simulink model "general_charger_2_cc_cv_test"  (R2013a)
settings: Solver=ode23  StartTime=0  StopTime=1.5  RelTol=1e-3
PreLoadFcn:
  | Ts =5e-6;
values from neighbouring files (symbols this model uses):
  ac_volt = 169    [charger_init.m]    (also in charger_init_simpl.m)
  acdc_on_time = 0.2    [charger_init.m]    (also in charger_init_simpl.m = 0)
  Cdc = 2e-3    (= 0.002)    [charger_init.m]    (also in charger_init_simpl.m)
  dcAd = dcinvexp*(eye(dcnstates) + (Ts/2)*dcAc)    [charger_init.m]    (also in charger_init_simpl.m)
  dcBd = dcinvexp*dcBc    [charger_init.m]    (also in charger_init_simpl.m)
  dcCd = dcCc*dcinvexp*Ts    [charger_init.m]    (also in charger_init_simpl.m)
  dcDd = dcCc*dcinvexp*dcBc*(Ts/2) + dcDc    [charger_init.m]    (also in charger_init_simpl.m)
  ESLCd = 0.1e-9    (= 1e-10)    [charger_init.m]    (also in charger_init_simpl.m)
  ESRCd = 70e-3    (= 0.07)    [charger_init.m]    (also in charger_init_simpl.m)
  ESRLdcdc = 0.1    [charger_init.m]    (also in charger_init_simpl.m)
  ESRLin = 0.2    [charger_init.m]    (also in charger_init_simpl.m = 0.1)
  Ldcdc = 1.3e-3    (= 0.0013)    [charger_init.m]    (also in charger_init_simpl.m = 0.0014)
  Lin = 1.5e-3    (= 0.0015)    [charger_init.m]    (also in charger_init_simpl.m = 0.001)
  P = 1.92e3    (= 1920)    [charger_init.m]    (also in charger_init_simpl.m)
  Q = 0    [charger_init.m]    (also in charger_init_simpl.m)
  ramp = (dc_volt - Vdcmin)/(acdc_ramp_end_time)    (= 202)    [charger_init.m]    (also in charger_init_simpl.m = (dc_volt - Vdcmin)/(acdc_ramp_end_time))
  Rbatt = 0.20    (= 0.2)    [charger_init.m]    (also in charger_init_simpl.m = 0.1)
  switch_Ts = 5e-5    (= 5e-05)    [charger_init.m]    (also in charger_init_simpl.m)
  sys_Ts = 5e-6    (= 5e-06)    [charger_init.m]    (also in charger_init_simpl.m)
  Vdcmin = ac_volt + 10    (= 179)    [charger_init.m]    (also in charger_init_simpl.m)
  voc = 105    [charger_init.m]    (also in charger_init_simpl.m)
undefined symbols (not defined in the file or in its folder): CESR, cpi
undefined symbols (not defined in the file): active_power_on, Ad, Bd, Cd, dc_volt, dcdc_cc_ref, dcdc_cv_ref, dcdc_iki, dcdc_ikp, dcdc_on, dcdc_vki, dcdc_vkp, Dd, dq_id_ki, dq_id_kp, dq_iq_ki, dq_iq_kp, dq_vdc_ki, dq_vdc_kp, dqQ_ki, dqQ_kp, P_ki, P_kp, pi_iac_ki, pi_iac_kp, pi_vdc_ki, pi_vdc_kp, piQ_ki, piQ_kp, pr_iac_kp, pr_pr_ki, pr_pr_kp, pr_vdc_ki, pr_vdc_kp, reactive_power_on
libraries: simulink_extras x165, powerlib x61, simulink x35, powerlib_meascontrol x11
(part 3 of 7)

== system general_charger_2_cc_cv_test/control_stage/AC//DC Control/PR Controller ==
  inputs : Inport
  Add2 : Sum  Inputs=-+
  Add3 : Sum  Inputs=+-
  Constant2 : Constant  Value=vdc_ref
  Constant3 : Constant  Value=ac_peak
  Demux1 : Demux  Outputs=3
  Divide1 : Product  Inputs=/*
  PI Reactive Power Controller : Subsystem
  PI2 : Subsystem  mask{ki=vdc_ki, kp=vdc_kp, Ts_pi=Ts, int_sat_up=500, int_sat_low=-500, pi_sat_up=500, pi_sat_low=-500}
      mask prompts: ki "Integral Gain"; kp "Proportional Gain"; Ts_pi "Sample Time"; int_sat_up "Integral Saturation Upper"; int_sat_low "Integral Saturation Lower"; pi_sat_up "PI Controller Saturation Upper"; pi_sat_low "PI Controller Saturation Lower"
      mask Display: disp('PI')
  PR Controller : Subsystem
  Product2 : Product  RndMeth=Zero
  Scope : Scope  NumInputPorts=2
      settings: YMin=-1~-1  YMax=1~1  SaveName=ScopeData4
  Step1 : Step  Time=1/60  Before=1  After=0  SampleTime=0
  Switch3 : Switch  Threshold=0.5
  v_cont : Outport
  wires:
  Constant2/1 -> Add2/2
  Demux1/2 -> Add2/1  "vdc"
  Add2/1 -> PI2/1(in)
  PI2/1(out) -> Product2/2
  Demux1/1 -> Divide1/2  "vac"
  Constant3/1 -> Divide1/1
  Product2/1 -> Add3/1
  Demux1/3 -> Add3/2  "iac"
  Add3/1 -> PR Controller/2(iac error)
  PR Controller/1(output) -> v_cont/1
  Divide1/1 -> Switch3/1, PI Reactive Power Controller/1(vac in)
  PI Reactive Power Controller/1(vac shifted) -> Switch3/3
  Step1/1 -> Switch3/2
  inputs/1 -> Demux1/1
  Switch3/1 -> Product2/1, PR Controller/1(vac)

== system general_charger_2_cc_cv_test/control_stage/DC//DC Control/DC Pass Filter (1st Order)1 ==
  u[k] : Inport
  A : Gain  Gain=dcAd
  B : Gain  Gain=dcBd
  C : Gain  Gain=dcCd
  D : Gain  Gain=dcDd
  Delay : Delay  DelayLength=1  InitialCondition=0  SampleTime=5e-5
  Sum : Sum  Inputs=|++
  Sum1 : Sum  Inputs=|++
  y[k] : Outport
  wires:
  B/1 -> Sum/1
  u[k]/1 -> D/1, B/1
  Sum1/1 -> y[k]/1
  Delay/1 -> A/1, C/1
  Sum/1 -> Delay/1
  D/1 -> Sum1/1
  A/1 -> Sum/2
  C/1 -> Sum1/2

== system general_charger_2_cc_cv_test/control_stage/DC//DC Control/PI1 ==
  in : Inport
  Add1 : Sum
  Add2 : Sum
  Constant : Constant  Value=0
  Ki : Gain  Gain=ki
  Kp : Gain  Gain=kp
  Step : Step  Time=pi_on  SampleTime=0
  Switch : Switch  Threshold=0.5
  Tappe : simulink/Discrete/Tapped Delay  vinit=0.0  samptime=Ts_pi  NumDelays=1  DelayOrder=Oldest  includeCurrent=off
  Ts : Gain  Gain=Ts_pi
  integral saturation : Saturate  UpperLimit=int_sat_up  LowerLimit=int_sat_low  SampleTime=Ts_pi
  pi controller saturation : Saturate  UpperLimit=pi_sat_up  LowerLimit=pi_sat_low  SampleTime=Ts_pi
  out : Outport
  wires:
  Ts/1 -> Ki/1
  Add1/1 -> integral saturation/1  "vdc_int_pi"
  Kp/1 -> Add2/2  "vdc_kp_pi"
  pi controller saturation/1 -> out/1
  Tappe/1 -> Add1/1
  Ki/1 -> Add1/2
  integral saturation/1 -> Add2/1, Tappe/1
  Step/1 -> Switch/2
  Constant/1 -> Switch/3
  Add2/1 -> pi controller saturation/1  "vdc_pi"
  Switch/1 -> Kp/1, Ts/1
  in/1 -> Switch/1  "vdc_error"

== system general_charger_2_cc_cv_test/control_stage/DC//DC Control/PI2 ==
  in : Inport
  Add1 : Sum
  Add2 : Sum
  Constant : Constant  Value=0
  Constant1 : Constant  Value=0
  Ki : Gain  Gain=ki
  Kp : Gain  Gain=kp
  Logical Operator : Logic  Operator=XOR  IconShape=distinctive  AllPortsSameDT=off  OutDataTypeStr=boolean
  Scope : Scope
      settings: SaveName=ScopeData21
  Step : Step  Time=pi_on  SampleTime=0
  Step1 : Step  Time=pturn_on  SampleTime=switch_Ts
  Step2 : Step  Time=pturn_on + switch_Ts  SampleTime=switch_Ts
  Switch : Switch  Threshold=0.5
  Switch1 : Switch  Threshold=0.5
  Tappe : simulink/Discrete/Tapped Delay  vinit=0.0  samptime=Ts_pi  NumDelays=1  DelayOrder=Oldest  includeCurrent=off
  Ts : Gain  Gain=Ts_pi
  integral saturation : Saturate  UpperLimit=int_sat_up  LowerLimit=int_sat_low  SampleTime=Ts_pi
  pi controller saturation : Saturate  UpperLimit=pi_sat_up  LowerLimit=pi_sat_low  SampleTime=Ts_pi
  out : Outport
  wires:
  Ts/1 -> Ki/1
  Add1/1 -> integral saturation/1  "vdc_int_pi"
  Kp/1 -> Add2/2  "vdc_kp_pi"
  pi controller saturation/1 -> out/1
  Ki/1 -> Add1/2
  integral saturation/1 -> Add2/1, Tappe/1
  Step/1 -> Switch/2
  Constant/1 -> Switch/3
  Add2/1 -> pi controller saturation/1  "vdc_pi"
  Switch/1 -> Kp/1, Ts/1
  in/1 -> Switch/1  "vdc_error"
  Tappe/1 -> Switch1/3
  Switch1/1 -> Add1/1
  Logical Operator/1 -> Switch1/2, Scope/1
  Step2/1 -> Logical Operator/2
  Step1/1 -> Logical Operator/1
  Constant1/1 -> Switch1/1

== system general_charger_2_cc_cv_test/control_stage/DC//DC Control/PI3 ==
  in : Inport
  Add1 : Sum
  Add2 : Sum
  Constant : Constant  Value=0
  Ki : Gain  Gain=ki
  Kp : Gain  Gain=kp
  Step : Step  Time=pi_on  SampleTime=0
  Switch : Switch  Threshold=0.5
  Tappe : simulink/Discrete/Tapped Delay  vinit=0.0  samptime=Ts_pi  NumDelays=1  DelayOrder=Oldest  includeCurrent=off
  Ts : Gain  Gain=Ts_pi
  integral saturation : Saturate  UpperLimit=int_sat_up  LowerLimit=int_sat_low  SampleTime=Ts_pi
  pi controller saturation : Saturate  UpperLimit=pi_sat_up  LowerLimit=pi_sat_low  SampleTime=Ts_pi
  out : Outport
  wires:
  Ts/1 -> Ki/1
  Add1/1 -> integral saturation/1  "vdc_int_pi"
  Kp/1 -> Add2/2  "vdc_kp_pi"
  pi controller saturation/1 -> out/1
  Tappe/1 -> Add1/1
  Ki/1 -> Add1/2
  integral saturation/1 -> Add2/1, Tappe/1
  Step/1 -> Switch/2
  Constant/1 -> Switch/3
  Add2/1 -> pi controller saturation/1  "vdc_pi"
  Switch/1 -> Kp/1, Ts/1
  in/1 -> Switch/1  "vdc_error"

== system general_charger_2_cc_cv_test/control_stage/DC//DC Control/PI4 ==
  in : Inport
  Add1 : Sum
  Add2 : Sum
  Constant : Constant  Value=0
  Ki : Gain  Gain=ki
  Kp : Gain  Gain=kp
  Step : Step  Time=pi_on  SampleTime=0
  Switch : Switch  Threshold=0.5
  Tappe : simulink/Discrete/Tapped Delay  vinit=0.0  samptime=Ts_pi  NumDelays=1  DelayOrder=Oldest  includeCurrent=off
  Ts : Gain  Gain=Ts_pi
  integral saturation : Saturate  UpperLimit=int_sat_up  LowerLimit=int_sat_low  SampleTime=Ts_pi
  pi controller saturation : Saturate  UpperLimit=pi_sat_up  LowerLimit=pi_sat_low  SampleTime=Ts_pi
  out : Outport
  wires:
  Ts/1 -> Ki/1
  Add1/1 -> integral saturation/1  "vdc_int_pi"
  Kp/1 -> Add2/2  "vdc_kp_pi"
  pi controller saturation/1 -> out/1
  Tappe/1 -> Add1/1
  Ki/1 -> Add1/2
  integral saturation/1 -> Add2/1, Tappe/1
  Step/1 -> Switch/2
  Constant/1 -> Switch/3
  Add2/1 -> pi controller saturation/1  "vdc_pi"
  Switch/1 -> Kp/1, Ts/1
  in/1 -> Switch/1  "vdc_error"

== system general_charger_2_cc_cv_test/control_stage/DC//DC Control/half bridge control ==
  v_cont : Inport
  Add1 : Sum
  Constant : Constant
  Constant1 : Constant  Value=0
  Constant2 : Constant  Value=2500
  Constant3 : Constant  Value=0
  Logical Operator : Logic  Operator=NOT  IconShape=distinctive  AllPortsSameDT=off  OutDataTypeStr=boolean
  Product2 : Product  RndMeth=Zero
  Relational Operator1 : RelationalOperator  OutDataTypeStr=boolean
  Repeating Sequence2 : simulink/Sources/Repeating Sequence  rep_seq_t=[0 25e-6 50e-6]  rep_seq_y=[0 2500 0]
  Saturation1 : Saturate  UpperLimit=2500  LowerLimit=0
  Step : Step  Time=turn_on  SampleTime=0
  Step1 : Step  Time=turn_on  SampleTime=0
  Switch : Switch  Threshold=0.5
  Switch1 : Switch  Threshold=0.5
  tag scope: E=global, F=global
  wires:
  v_cont/1 -> Product2/2
  Repeating Sequence2/1 -> Relational Operator1/2
  Constant2/1 -> Product2/1
  Saturation1/1 -> Relational Operator1/1
  Product2/1 -> Add1/2
  Constant1/1 -> Add1/1
  Add1/1 -> Saturation1/1
  Logical Operator/1 -> [F]
  Step/1 -> Switch/2
  Constant/1 -> Switch/3
  Step1/1 -> Switch1/2
  Constant3/1 -> Switch1/3
  Relational Operator1/1 -> Switch/1, Switch1/1
  Switch/1 -> Logical Operator/1
  Switch1/1 -> [E]

== system general_charger_2_cc_cv_test/Measurements/Power and angle calculations/AB-DQ Transform/Iab_dq ==
  A : Inport
  wt : Inport  Port=2
  phi : Inport  Port=3
  Add1 : Sum  Inputs=-+
  Add2 : Sum
  Delay : Delay  DelayLength=RSpC  SampleTime=abdq_Ts
  Gain : Gain  Gain=-1
  Id Discretization Error Correction : Subsystem
  Iq Discretization Error Correction : Subsystem
  Product{1..4} (4 alike) : Product  RndMeth=Zero
  Scope : Scope  NumInputPorts=4
      settings: YMin=3.5~3.5~-17.5~-17.5  YMax=10~10~2.5~2.5  SaveName=ScopeData13
  Trigonometric Function : Trigonometry
  Trigonometric Function1 : Trigonometry  Operator=cos
  Unit Delay : UnitDelay  SampleTime=switch_Ts
  D : Outport
  Q : Outport  Port=2
  wires:
  Trigonometric Function/1 -> Product1/1, Product2/1
  Product1/1 -> Add2/2
  Product4/1 -> Add2/1
  Product2/1 -> Add1/1
  A/1 -> Delay/1, Product4/1, Product2/2
  Trigonometric Function1/1 -> Product4/2, Product3/1
  Product3/1 -> Add1/2
  Delay/1 -> Product1/2, Product3/2  "B"
  wt/1 -> [theta], Trigonometric Function1/1, Trigonometric Function/1
  Add2/1 -> Scope/2, Id Discretization Error Correction/3(D)  "Vd"
  Add1/1 -> Scope/3, Iq Discretization Error Correction/2(Q)
  [theta] -> Iq Discretization Error Correction/3(wt)
  [theta] -> Id Discretization Error Correction/2(wt)
  Id Discretization Error Correction/1(Id_corr) -> Scope/1, D/1
  Iq Discretization Error Correction/1(Iq_corr) -> Scope/4, Q/1
  phi/1 -> Gain/1
  Unit Delay/1 -> Iq Discretization Error Correction/1(phi), Id Discretization Error Correction/4(phi)
  Gain/1 -> Unit Delay/1
  [Ipeak] -> Iq Discretization Error Correction/4(A)
  [Ipeak] -> Id Discretization Error Correction/1(A)

== system general_charger_2_cc_cv_test/Measurements/Power and angle calculations/AB-DQ Transform/Vab_dq ==
  note: PLL based on dq frame control
      | input signal is assumed to be 60 Hz
      | and sample time is 50e-6
  signal_in : Inport
  AB->DQ : Subsystem  mask{abdq_f=pll_f, abdq_Ts=pll_Ts}
      mask prompts: abdq_f "frequency"; abdq_Ts "Sample Time"
      mask init:
      | SpC=1/abdq_f/4/abdq_Ts;
      | RSpC=ceil(SpC);
  Constant1 : Constant  Value=0
  Constant3 : Constant  Value=2*pi*pll_f
  PI1 : Subsystem  mask{ki=1, kp=0, Ts_pi=pll_Ts, int_sat_up=inf, int_sat_low=-inf, pi_sat_up=inf, pi_sat_low=-inf}
      mask prompts: ki "Integral Gain"; kp "Proportional Gain"; Ts_pi "Sample Time"; int_sat_up "Integral Saturation Upper"; int_sat_low "Integral Saturation Lower"; pi_sat_up "PI Controller Saturation Upper"; pi_sat_low "PI Controller Saturation Lower"
      mask Display: disp('PI')
  PI4 : Subsystem  mask{ki=pll_ki, kp=pll_kp, Ts_pi=pll_Ts, int_sat_up=inf, int_sat_low=-inf, pi_sat_up=inf, pi_sat_low=-inf}
      mask prompts: ki "Integral Gain"; kp "Proportional Gain"; Ts_pi "Sample Time"; int_sat_up "Integral Saturation Upper"; int_sat_low "Integral Saturation Lower"; pi_sat_up "PI Controller Saturation Upper"; pi_sat_low "PI Controller Saturation Lower"
      mask Display: disp('PI')
  Sum : Sum  Inputs=|-+
  Sum2 : Sum  Inputs=|-+
  angle_out : Outport
  D : Outport  Port=2
  Q : Outport  Port=3
  wires:
  Constant1/1 -> Sum/2
  Sum/1 -> PI4/1(in)
  PI1/1(out) -> angle_out/1, AB->DQ/2(wt)
  Constant3/1 -> Sum2/2
  PI4/1(out) -> Sum2/1
  AB->DQ/2(Q) -> Q/1, Sum/1
  signal_in/1 -> AB->DQ/1(A)
  AB->DQ/1(D) -> D/1
  Sum2/1 -> PI1/1(in)  "pll_int_error"

== system general_charger_2_cc_cv_test/Measurements/Power and angle calculations/RMS1/PI3 ==
  in : Inport
  Add1 : Sum
  Add2 : Sum
  Ki : Gain  Gain=ki
  Kp : Gain  Gain=kp
  Tappe : simulink/Discrete/Tapped Delay  vinit=0.0  samptime=Ts_pi  NumDelays=1  DelayOrder=Oldest  includeCurrent=off
  Ts : Gain  Gain=Ts_pi
  integral saturation : Saturate  UpperLimit=int_sat_up  LowerLimit=int_sat_low  SampleTime=Ts_pi
  pi controller saturation : Saturate  UpperLimit=pi_sat_up  LowerLimit=pi_sat_low  SampleTime=Ts_pi
  out : Outport
  wires:
  Ts/1 -> Ki/1
  in/1 -> Kp/1, Ts/1  "vdc_error"
  Add1/1 -> integral saturation/1  "vdc_int_pi"
  Kp/1 -> Add2/2  "vdc_kp_pi"
  pi controller saturation/1 -> out/1
  Tappe/1 -> Add1/1
  Add2/1 -> pi controller saturation/1  "vdc_pi"
  Ki/1 -> Add1/2
  integral saturation/1 -> Add2/1, Tappe/1

== system general_charger_2_cc_cv_test/Measurements/Power and angle calculations/RMS4/PI3 ==
  in : Inport
  Add1 : Sum
  Add2 : Sum
  Ki : Gain  Gain=ki
  Kp : Gain  Gain=kp
  Tappe : simulink/Discrete/Tapped Delay  vinit=0.0  samptime=Ts_pi  NumDelays=1  DelayOrder=Oldest  includeCurrent=off
  Ts : Gain  Gain=Ts_pi
  integral saturation : Saturate  UpperLimit=int_sat_up  LowerLimit=int_sat_low  SampleTime=Ts_pi
  pi controller saturation : Saturate  UpperLimit=pi_sat_up  LowerLimit=pi_sat_low  SampleTime=Ts_pi
  out : Outport
  wires:
  Ts/1 -> Ki/1
  in/1 -> Kp/1, Ts/1  "vdc_error"
  Add1/1 -> integral saturation/1  "vdc_int_pi"
  Kp/1 -> Add2/2  "vdc_kp_pi"
  pi controller saturation/1 -> out/1
  Tappe/1 -> Add1/1
  Add2/1 -> pi controller saturation/1  "vdc_pi"
  Ki/1 -> Add1/2
  integral saturation/1 -> Add2/1, Tappe/1

== system general_charger_2_cc_cv_test/Measurements/Power and angle calculations/discrete low pass filter1/Ad(1,1) ==
  in : Inport
  Constant1 : Constant  Value=variable
  Product1 : Product
  q rounder16 : Subsystem  mask{q=nQ, range=maxRange}
      mask prompts: q "q value"; range "q range"
  out : Outport
  wires:
  q rounder16/1(out) -> Product1/1
  Constant1/1 -> q rounder16/1(in)
  Product1/1 -> out/1
  in/1 -> Product1/2

== system general_charger_2_cc_cv_test/Measurements/Power and angle calculations/discrete low pass filter1/Ad(1,2) ==
  in : Inport
  Constant1 : Constant  Value=variable
  Product1 : Product
  q rounder16 : Subsystem  mask{q=nQ, range=maxRange}
      mask prompts: q "q value"; range "q range"
  out : Outport
  wires:
  q rounder16/1(out) -> Product1/1
  Constant1/1 -> q rounder16/1(in)
  Product1/1 -> out/1
  in/1 -> Product1/2

== system general_charger_2_cc_cv_test/Measurements/Power and angle calculations/discrete low pass filter1/Ad(1,3) ==
  in : Inport
  Constant1 : Constant  Value=variable
  Product1 : Product
  Scope1 : Scope  NumInputPorts=2
      settings: YMin=-5~-5  YMax=5~5
  q rounder16 : Subsystem  mask{q=nQ, range=maxRange}
      mask prompts: q "q value"; range "q range"
  out : Outport
  wires:
  q rounder16/1(out) -> Product1/1, Scope1/2
  Constant1/1 -> Scope1/1, q rounder16/1(in)
  Product1/1 -> out/1
  in/1 -> Product1/2

== system general_charger_2_cc_cv_test/Measurements/Power and angle calculations/discrete low pass filter1/Ad(2,1) ==
  in : Inport
  Constant1 : Constant  Value=variable
  Product1 : Product
  Scope1 : Scope  NumInputPorts=2
      settings: YMin=-5~-5  YMax=5~5
  q rounder16 : Subsystem  mask{q=nQ, range=maxRange}
      mask prompts: q "q value"; range "q range"
  out : Outport
  wires:
  q rounder16/1(out) -> Product1/1, Scope1/2
  Constant1/1 -> Scope1/1, q rounder16/1(in)
  Product1/1 -> out/1
  in/1 -> Product1/2

== system general_charger_2_cc_cv_test/Measurements/Power and angle calculations/discrete low pass filter1/Ad(2,2) ==
  in : Inport
  Constant1 : Constant  Value=variable
  Product1 : Product
  Scope1 : Scope  NumInputPorts=2
      settings: YMin=-5~-5  YMax=5~5
  q rounder16 : Subsystem  mask{q=nQ, range=maxRange}
      mask prompts: q "q value"; range "q range"
  out : Outport
  wires:
  q rounder16/1(out) -> Product1/1, Scope1/2
  Constant1/1 -> Scope1/1, q rounder16/1(in)
  Product1/1 -> out/1
  in/1 -> Product1/2

== system general_charger_2_cc_cv_test/Measurements/Power and angle calculations/discrete low pass filter1/Ad(2,3) ==
  in : Inport
  Constant1 : Constant  Value=variable
  Product1 : Product
  Scope1 : Scope  NumInputPorts=2
      settings: YMin=-5~-5  YMax=5~5
  q rounder16 : Subsystem  mask{q=nQ, range=maxRange}
      mask prompts: q "q value"; range "q range"
  out : Outport
  wires:
  q rounder16/1(out) -> Product1/1, Scope1/2
  Constant1/1 -> Scope1/1, q rounder16/1(in)
  Product1/1 -> out/1
  in/1 -> Product1/2

== system general_charger_2_cc_cv_test/Measurements/Power and angle calculations/discrete low pass filter1/Ad(3,1) ==
  in : Inport
  Constant1 : Constant  Value=variable
  Product1 : Product
  Scope1 : Scope  NumInputPorts=2
      settings: YMin=-5~-5  YMax=5~5
  q rounder16 : Subsystem  mask{q=nQ, range=maxRange}
      mask prompts: q "q value"; range "q range"
  out : Outport
  wires:
  q rounder16/1(out) -> Product1/1, Scope1/2
  Constant1/1 -> Scope1/1, q rounder16/1(in)
  Product1/1 -> out/1
  in/1 -> Product1/2

== system general_charger_2_cc_cv_test/Measurements/Power and angle calculations/discrete low pass filter1/Ad(3,2) ==
  in : Inport
  Constant1 : Constant  Value=variable
  Product1 : Product
  Scope1 : Scope  NumInputPorts=2
      settings: YMin=-5~-5  YMax=5~5
  q rounder16 : Subsystem  mask{q=nQ, range=maxRange}
      mask prompts: q "q value"; range "q range"
  out : Outport
  wires:
  q rounder16/1(out) -> Product1/1, Scope1/2
  Constant1/1 -> Scope1/1, q rounder16/1(in)
  Product1/1 -> out/1
  in/1 -> Product1/2

== system general_charger_2_cc_cv_test/Measurements/Power and angle calculations/discrete low pass filter1/Ad(3,3) ==
  in : Inport
  Constant1 : Constant  Value=variable
  Product1 : Product
  Scope1 : Scope  NumInputPorts=2
      settings: YMin=-5~-5  YMax=5~5
  q rounder16 : Subsystem  mask{q=nQ, range=maxRange}
      mask prompts: q "q value"; range "q range"
  out : Outport
  wires:
  q rounder16/1(out) -> Product1/1, Scope1/2
  Constant1/1 -> Scope1/1, q rounder16/1(in)
  Product1/1 -> out/1
  in/1 -> Product1/2

== system general_charger_2_cc_cv_test/Measurements/Power and angle calculations/discrete low pass filter1/Bd(1) ==
  in : Inport
  Constant1 : Constant  Value=variable
  Product1 : Product
  q rounder16 : Subsystem  mask{q=nQ, range=maxRange}
      mask prompts: q "q value"; range "q range"
  out : Outport
  wires:
  q rounder16/1(out) -> Product1/1
  Constant1/1 -> q rounder16/1(in)
  Product1/1 -> out/1
  in/1 -> Product1/2

== system general_charger_2_cc_cv_test/Measurements/Power and angle calculations/discrete low pass filter1/Bd(2) ==
  in : Inport
  Constant1 : Constant  Value=variable
  Product1 : Product
  q rounder16 : Subsystem  mask{q=nQ, range=maxRange}
      mask prompts: q "q value"; range "q range"
  out : Outport
  wires:
  q rounder16/1(out) -> Product1/1
  Constant1/1 -> q rounder16/1(in)
  Product1/1 -> out/1
  in/1 -> Product1/2

== system general_charger_2_cc_cv_test/Measurements/Power and angle calculations/discrete low pass filter1/Bd(3) ==
  in : Inport
  Constant1 : Constant  Value=variable
  Product1 : Product
  q rounder16 : Subsystem  mask{q=nQ, range=maxRange}
      mask prompts: q "q value"; range "q range"
  out : Outport
  wires:
  q rounder16/1(out) -> Product1/1
  Constant1/1 -> q rounder16/1(in)
  Product1/1 -> out/1
  in/1 -> Product1/2

== system general_charger_2_cc_cv_test/Measurements/Power and angle calculations/discrete low pass filter1/Cd(1) ==
  in : Inport
  Constant1 : Constant  Value=variable
  Product1 : Product
  q rounder16 : Subsystem  mask{q=nQ, range=maxRange}
      mask prompts: q "q value"; range "q range"
  out : Outport
  wires:
  q rounder16/1(out) -> Product1/1
  Constant1/1 -> q rounder16/1(in)
  Product1/1 -> out/1
  in/1 -> Product1/2

== system general_charger_2_cc_cv_test/Measurements/Power and angle calculations/discrete low pass filter1/Cd(2) ==
  in : Inport
  Constant1 : Constant  Value=variable
  Product1 : Product
  q rounder16 : Subsystem  mask{q=nQ, range=maxRange}
      mask prompts: q "q value"; range "q range"
  out : Outport
  wires:
  q rounder16/1(out) -> Product1/1
  Constant1/1 -> q rounder16/1(in)
  Product1/1 -> out/1
  in/1 -> Product1/2

== system general_charger_2_cc_cv_test/Measurements/Power and angle calculations/discrete low pass filter1/Cd(3) ==
  in : Inport
  Constant1 : Constant  Value=variable
  Product1 : Product
  q rounder16 : Subsystem  mask{q=nQ, range=maxRange}
      mask prompts: q "q value"; range "q range"
  out : Outport
  wires:
  q rounder16/1(out) -> Product1/1
  Constant1/1 -> q rounder16/1(in)
  Product1/1 -> out/1
  in/1 -> Product1/2

== system general_charger_2_cc_cv_test/Measurements/Power and angle calculations/discrete low pass filter1/Dd ==
  in : Inport
  Constant1 : Constant  Value=variable
  Product1 : Product
  Scope1 : Scope  NumInputPorts=2
      settings: YMin=-5~-5  YMax=5~5
  q rounder16 : Subsystem  mask{q=nQ, range=maxRange}
      mask prompts: q "q value"; range "q range"
  out : Outport
  wires:
  q rounder16/1(out) -> Product1/1, Scope1/2
  Constant1/1 -> Scope1/1, q rounder16/1(in)
  Product1/1 -> out/1
  in/1 -> Product1/2

== system general_charger_2_cc_cv_test/Measurements/Power and angle calculations/discrete low pass filter1/q rounder1 ==
  in : Inport
  Gain9 : Gain  Gain=2^-q
  Idealized ADC quantizer : simulink_extras/Additional Discrete/Idealized ADC quantizer  NumberOfConverterBits=32  Vmin=-range  Vmax=range  OutputDataType=double  OutputNegativeValues=on
  out : Outport
  wires:
  in/1 -> Idealized ADC quantizer/1
  Idealized ADC quantizer/1 -> Gain9/1
  Gain9/1 -> out/1

== system general_charger_2_cc_cv_test/Measurements/Power and angle calculations/discrete low pass filter1/q rounder10 ==
  in : Inport
  Gain9 : Gain  Gain=2^-q
  Idealized ADC quantizer : simulink_extras/Additional Discrete/Idealized ADC quantizer  NumberOfConverterBits=32  Vmin=-range  Vmax=range  OutputDataType=double  OutputNegativeValues=on
  out : Outport
  wires:
  in/1 -> Idealized ADC quantizer/1
  Idealized ADC quantizer/1 -> Gain9/1
  Gain9/1 -> out/1

== system general_charger_2_cc_cv_test/Measurements/Power and angle calculations/discrete low pass filter1/q rounder11 ==
  in : Inport
  Gain9 : Gain  Gain=2^-q
  Idealized ADC quantizer : simulink_extras/Additional Discrete/Idealized ADC quantizer  NumberOfConverterBits=32  Vmin=-range  Vmax=range  OutputDataType=double  OutputNegativeValues=on
  out : Outport
  wires:
  in/1 -> Idealized ADC quantizer/1
  Idealized ADC quantizer/1 -> Gain9/1
  Gain9/1 -> out/1

== system general_charger_2_cc_cv_test/Measurements/Power and angle calculations/discrete low pass filter1/q rounder12 ==
  in : Inport
  Gain9 : Gain  Gain=2^-q
  Idealized ADC quantizer : simulink_extras/Additional Discrete/Idealized ADC quantizer  NumberOfConverterBits=32  Vmin=-range  Vmax=range  OutputDataType=double  OutputNegativeValues=on
  out : Outport
  wires:
  in/1 -> Idealized ADC quantizer/1
  Idealized ADC quantizer/1 -> Gain9/1
  Gain9/1 -> out/1

== system general_charger_2_cc_cv_test/Measurements/Power and angle calculations/discrete low pass filter1/q rounder13 ==
  in : Inport
  Gain9 : Gain  Gain=2^-q
  Idealized ADC quantizer : simulink_extras/Additional Discrete/Idealized ADC quantizer  NumberOfConverterBits=32  Vmin=-range  Vmax=range  OutputDataType=double  OutputNegativeValues=on
  out : Outport
  wires:
  in/1 -> Idealized ADC quantizer/1
  Idealized ADC quantizer/1 -> Gain9/1
  Gain9/1 -> out/1

== system general_charger_2_cc_cv_test/Measurements/Power and angle calculations/discrete low pass filter1/q rounder14 ==
  in : Inport
  Gain9 : Gain  Gain=2^-q
  Idealized ADC quantizer : simulink_extras/Additional Discrete/Idealized ADC quantizer  NumberOfConverterBits=32  Vmin=-range  Vmax=range  OutputDataType=double  OutputNegativeValues=on
  out : Outport
  wires:
  in/1 -> Idealized ADC quantizer/1
  Idealized ADC quantizer/1 -> Gain9/1
  Gain9/1 -> out/1

== system general_charger_2_cc_cv_test/Measurements/Power and angle calculations/discrete low pass filter1/q rounder15 ==
  in : Inport
  Gain9 : Gain  Gain=2^-q
  Idealized ADC quantizer : simulink_extras/Additional Discrete/Idealized ADC quantizer  NumberOfConverterBits=32  Vmin=-range  Vmax=range  OutputDataType=double  OutputNegativeValues=on
  out : Outport
  wires:
  in/1 -> Idealized ADC quantizer/1
  Idealized ADC quantizer/1 -> Gain9/1
  Gain9/1 -> out/1

== system general_charger_2_cc_cv_test/Measurements/Power and angle calculations/discrete low pass filter1/q rounder16 ==
  in : Inport
  Gain9 : Gain  Gain=2^-q
  Idealized ADC quantizer : simulink_extras/Additional Discrete/Idealized ADC quantizer  NumberOfConverterBits=32  Vmin=-range  Vmax=range  OutputDataType=double  OutputNegativeValues=on
  out : Outport
  wires:
  in/1 -> Idealized ADC quantizer/1
  Idealized ADC quantizer/1 -> Gain9/1
  Gain9/1 -> out/1

== system general_charger_2_cc_cv_test/Measurements/Power and angle calculations/discrete low pass filter1/q rounder17 ==
  in : Inport
  Gain9 : Gain  Gain=2^-q
  Idealized ADC quantizer : simulink_extras/Additional Discrete/Idealized ADC quantizer  NumberOfConverterBits=32  Vmin=-range  Vmax=range  OutputDataType=double  OutputNegativeValues=on
  out : Outport
  wires:
  in/1 -> Idealized ADC quantizer/1
  Idealized ADC quantizer/1 -> Gain9/1
  Gain9/1 -> out/1

== system general_charger_2_cc_cv_test/Measurements/Power and angle calculations/discrete low pass filter1/q rounder2 ==
  in : Inport
  Gain9 : Gain  Gain=2^-q
  Idealized ADC quantizer : simulink_extras/Additional Discrete/Idealized ADC quantizer  NumberOfConverterBits=32  Vmin=-range  Vmax=range  OutputDataType=double  OutputNegativeValues=on
  out : Outport
  wires:
  in/1 -> Idealized ADC quantizer/1
  Idealized ADC quantizer/1 -> Gain9/1
  Gain9/1 -> out/1

== system general_charger_2_cc_cv_test/Measurements/Power and angle calculations/discrete low pass filter1/q rounder3 ==
  in : Inport
  Gain9 : Gain  Gain=2^-q
  Idealized ADC quantizer : simulink_extras/Additional Discrete/Idealized ADC quantizer  NumberOfConverterBits=32  Vmin=-range  Vmax=range  OutputDataType=double  OutputNegativeValues=on
  out : Outport
  wires:
  in/1 -> Idealized ADC quantizer/1
  Idealized ADC quantizer/1 -> Gain9/1
  Gain9/1 -> out/1

== system general_charger_2_cc_cv_test/Measurements/Power and angle calculations/discrete low pass filter1/q rounder4 ==
  in : Inport
  Gain9 : Gain  Gain=2^-q
  Idealized ADC quantizer : simulink_extras/Additional Discrete/Idealized ADC quantizer  NumberOfConverterBits=32  Vmin=-range  Vmax=range  OutputDataType=double  OutputNegativeValues=on
  out : Outport
  wires:
  in/1 -> Idealized ADC quantizer/1
  Idealized ADC quantizer/1 -> Gain9/1
  Gain9/1 -> out/1

== system general_charger_2_cc_cv_test/Measurements/Power and angle calculations/discrete low pass filter1/q rounder5 ==
  in : Inport
  Gain9 : Gain  Gain=2^-q
  Idealized ADC quantizer : simulink_extras/Additional Discrete/Idealized ADC quantizer  NumberOfConverterBits=32  Vmin=-range  Vmax=range  OutputDataType=double  OutputNegativeValues=on
  out : Outport
  wires:
  in/1 -> Idealized ADC quantizer/1
  Idealized ADC quantizer/1 -> Gain9/1
  Gain9/1 -> out/1

== system general_charger_2_cc_cv_test/Measurements/Power and angle calculations/discrete low pass filter1/q rounder6 ==
  in : Inport
  Gain9 : Gain  Gain=2^-q
  Idealized ADC quantizer : simulink_extras/Additional Discrete/Idealized ADC quantizer  NumberOfConverterBits=32  Vmin=-range  Vmax=range  OutputDataType=double  OutputNegativeValues=on
  out : Outport
  wires:
  in/1 -> Idealized ADC quantizer/1
  Idealized ADC quantizer/1 -> Gain9/1
  Gain9/1 -> out/1

== system general_charger_2_cc_cv_test/Measurements/Power and angle calculations/discrete low pass filter1/q rounder7 ==
  in : Inport
  Gain9 : Gain  Gain=2^-q
  Idealized ADC quantizer : simulink_extras/Additional Discrete/Idealized ADC quantizer  NumberOfConverterBits=32  Vmin=-range  Vmax=range  OutputDataType=double  OutputNegativeValues=on
  out : Outport
  wires:
  in/1 -> Idealized ADC quantizer/1
  Idealized ADC quantizer/1 -> Gain9/1
  Gain9/1 -> out/1

== system general_charger_2_cc_cv_test/Measurements/Power and angle calculations/discrete low pass filter1/q rounder8 ==
  in : Inport
  Gain9 : Gain  Gain=2^-q
  Idealized ADC quantizer : simulink_extras/Additional Discrete/Idealized ADC quantizer  NumberOfConverterBits=32  Vmin=-range  Vmax=range  OutputDataType=double  OutputNegativeValues=on
  out : Outport
  wires:
  in/1 -> Idealized ADC quantizer/1
  Idealized ADC quantizer/1 -> Gain9/1
  Gain9/1 -> out/1

== system general_charger_2_cc_cv_test/Measurements/Power and angle calculations/discrete low pass filter1/q rounder9 ==
  in : Inport
  Gain9 : Gain  Gain=2^-q
  Idealized ADC quantizer : simulink_extras/Additional Discrete/Idealized ADC quantizer  NumberOfConverterBits=32  Vmin=-range  Vmax=range  OutputDataType=double  OutputNegativeValues=on
  out : Outport
  wires:
  in/1 -> Idealized ADC quantizer/1
  Idealized ADC quantizer/1 -> Gain9/1
  Gain9/1 -> out/1

== system general_charger_2_cc_cv_test/Measurements/Power and angle calculations/discrete low pass filter2/Ad(1,1) ==
  in : Inport
  Constant1 : Constant  Value=variable
  Product1 : Product
  q rounder16 : Subsystem  mask{q=nQ, range=maxRange}
      mask prompts: q "q value"; range "q range"
  out : Outport
  wires:
  q rounder16/1(out) -> Product1/1
  Constant1/1 -> q rounder16/1(in)
  Product1/1 -> out/1
  in/1 -> Product1/2

== system general_charger_2_cc_cv_test/Measurements/Power and angle calculations/discrete low pass filter2/Ad(1,2) ==
  in : Inport
  Constant1 : Constant  Value=variable
  Product1 : Product
  q rounder16 : Subsystem  mask{q=nQ, range=maxRange}
      mask prompts: q "q value"; range "q range"
  out : Outport
  wires:
  q rounder16/1(out) -> Product1/1
  Constant1/1 -> q rounder16/1(in)
  Product1/1 -> out/1
  in/1 -> Product1/2

== system general_charger_2_cc_cv_test/Measurements/Power and angle calculations/discrete low pass filter2/Ad(1,3) ==
  in : Inport
  Constant1 : Constant  Value=variable
  Product1 : Product
  Scope1 : Scope  NumInputPorts=2
      settings: YMin=-5~-5  YMax=5~5
  q rounder16 : Subsystem  mask{q=nQ, range=maxRange}
      mask prompts: q "q value"; range "q range"
  out : Outport
  wires:
  q rounder16/1(out) -> Product1/1, Scope1/2
  Constant1/1 -> Scope1/1, q rounder16/1(in)
  Product1/1 -> out/1
  in/1 -> Product1/2

== system general_charger_2_cc_cv_test/Measurements/Power and angle calculations/discrete low pass filter2/Ad(2,1) ==
  in : Inport
  Constant1 : Constant  Value=variable
  Product1 : Product
  Scope1 : Scope  NumInputPorts=2
      settings: YMin=-5~-5  YMax=5~5
  q rounder16 : Subsystem  mask{q=nQ, range=maxRange}
      mask prompts: q "q value"; range "q range"
  out : Outport
  wires:
  q rounder16/1(out) -> Product1/1, Scope1/2
  Constant1/1 -> Scope1/1, q rounder16/1(in)
  Product1/1 -> out/1
  in/1 -> Product1/2

== system general_charger_2_cc_cv_test/Measurements/Power and angle calculations/discrete low pass filter2/Ad(2,2) ==
  in : Inport
  Constant1 : Constant  Value=variable
  Product1 : Product
  Scope1 : Scope  NumInputPorts=2
      settings: YMin=-5~-5  YMax=5~5
  q rounder16 : Subsystem  mask{q=nQ, range=maxRange}
      mask prompts: q "q value"; range "q range"
  out : Outport
  wires:
  q rounder16/1(out) -> Product1/1, Scope1/2
  Constant1/1 -> Scope1/1, q rounder16/1(in)
  Product1/1 -> out/1
  in/1 -> Product1/2

== system general_charger_2_cc_cv_test/Measurements/Power and angle calculations/discrete low pass filter2/Ad(2,3) ==
  in : Inport
  Constant1 : Constant  Value=variable
  Product1 : Product
  Scope1 : Scope  NumInputPorts=2
      settings: YMin=-5~-5  YMax=5~5
  q rounder16 : Subsystem  mask{q=nQ, range=maxRange}
      mask prompts: q "q value"; range "q range"
  out : Outport
  wires:
  q rounder16/1(out) -> Product1/1, Scope1/2
  Constant1/1 -> Scope1/1, q rounder16/1(in)
  Product1/1 -> out/1
  in/1 -> Product1/2

== system general_charger_2_cc_cv_test/Measurements/Power and angle calculations/discrete low pass filter2/Ad(3,1) ==
  in : Inport
  Constant1 : Constant  Value=variable
  Product1 : Product
  Scope1 : Scope  NumInputPorts=2
      settings: YMin=-5~-5  YMax=5~5
  q rounder16 : Subsystem  mask{q=nQ, range=maxRange}
      mask prompts: q "q value"; range "q range"
  out : Outport
  wires:
  q rounder16/1(out) -> Product1/1, Scope1/2
  Constant1/1 -> Scope1/1, q rounder16/1(in)
  Product1/1 -> out/1
  in/1 -> Product1/2

== system general_charger_2_cc_cv_test/Measurements/Power and angle calculations/discrete low pass filter2/Ad(3,2) ==
  in : Inport
  Constant1 : Constant  Value=variable
  Product1 : Product
  Scope1 : Scope  NumInputPorts=2
      settings: YMin=-5~-5  YMax=5~5
  q rounder16 : Subsystem  mask{q=nQ, range=maxRange}
      mask prompts: q "q value"; range "q range"
  out : Outport
  wires:
  q rounder16/1(out) -> Product1/1, Scope1/2
  Constant1/1 -> Scope1/1, q rounder16/1(in)
  Product1/1 -> out/1
  in/1 -> Product1/2

== system general_charger_2_cc_cv_test/Measurements/Power and angle calculations/discrete low pass filter2/Ad(3,3) ==
  in : Inport
  Constant1 : Constant  Value=variable
  Product1 : Product
  Scope1 : Scope  NumInputPorts=2
      settings: YMin=-5~-5  YMax=5~5
  q rounder16 : Subsystem  mask{q=nQ, range=maxRange}
      mask prompts: q "q value"; range "q range"
  out : Outport
  wires:
  q rounder16/1(out) -> Product1/1, Scope1/2
  Constant1/1 -> Scope1/1, q rounder16/1(in)
  Product1/1 -> out/1
  in/1 -> Product1/2

== system general_charger_2_cc_cv_test/Measurements/Power and angle calculations/discrete low pass filter2/Bd(1) ==
  in : Inport
  Constant1 : Constant  Value=variable
  Product1 : Product
  q rounder16 : Subsystem  mask{q=nQ, range=maxRange}
      mask prompts: q "q value"; range "q range"
  out : Outport
  wires:
  q rounder16/1(out) -> Product1/1
  Constant1/1 -> q rounder16/1(in)
  Product1/1 -> out/1
  in/1 -> Product1/2

== system general_charger_2_cc_cv_test/Measurements/Power and angle calculations/discrete low pass filter2/Bd(2) ==
  in : Inport
  Constant1 : Constant  Value=variable
  Product1 : Product
  q rounder16 : Subsystem  mask{q=nQ, range=maxRange}
      mask prompts: q "q value"; range "q range"
  out : Outport
  wires:
  q rounder16/1(out) -> Product1/1
  Constant1/1 -> q rounder16/1(in)
  Product1/1 -> out/1
  in/1 -> Product1/2

== system general_charger_2_cc_cv_test/Measurements/Power and angle calculations/discrete low pass filter2/Bd(3) ==
  in : Inport
  Constant1 : Constant  Value=variable
  Product1 : Product
  q rounder16 : Subsystem  mask{q=nQ, range=maxRange}
      mask prompts: q "q value"; range "q range"
  out : Outport
  wires:
  q rounder16/1(out) -> Product1/1
  Constant1/1 -> q rounder16/1(in)
  Product1/1 -> out/1
  in/1 -> Product1/2

== system general_charger_2_cc_cv_test/Measurements/Power and angle calculations/discrete low pass filter2/Cd(1) ==
  in : Inport
  Constant1 : Constant  Value=variable
  Product1 : Product
  q rounder16 : Subsystem  mask{q=nQ, range=maxRange}
      mask prompts: q "q value"; range "q range"
  out : Outport
  wires:
  q rounder16/1(out) -> Product1/1
  Constant1/1 -> q rounder16/1(in)
  Product1/1 -> out/1
  in/1 -> Product1/2

== system general_charger_2_cc_cv_test/Measurements/Power and angle calculations/discrete low pass filter2/Cd(2) ==
  in : Inport
  Constant1 : Constant  Value=variable
  Product1 : Product
  q rounder16 : Subsystem  mask{q=nQ, range=maxRange}
      mask prompts: q "q value"; range "q range"
  out : Outport
  wires:
  q rounder16/1(out) -> Product1/1
  Constant1/1 -> q rounder16/1(in)
  Product1/1 -> out/1
  in/1 -> Product1/2

== system general_charger_2_cc_cv_test/Measurements/Power and angle calculations/discrete low pass filter2/Cd(3) ==
  in : Inport
  Constant1 : Constant  Value=variable
  Product1 : Product
  q rounder16 : Subsystem  mask{q=nQ, range=maxRange}
      mask prompts: q "q value"; range "q range"
  out : Outport
  wires:
  q rounder16/1(out) -> Product1/1
  Constant1/1 -> q rounder16/1(in)
  Product1/1 -> out/1
  in/1 -> Product1/2

== system general_charger_2_cc_cv_test/Measurements/Power and angle calculations/discrete low pass filter2/Dd ==
  in : Inport
  Constant1 : Constant  Value=variable
  Product1 : Product
  Scope1 : Scope  NumInputPorts=2
      settings: YMin=-5~-5  YMax=5~5
  q rounder16 : Subsystem  mask{q=nQ, range=maxRange}
      mask prompts: q "q value"; range "q range"
  out : Outport
  wires:
  q rounder16/1(out) -> Product1/1, Scope1/2
  Constant1/1 -> Scope1/1, q rounder16/1(in)
  Product1/1 -> out/1
  in/1 -> Product1/2

== system general_charger_2_cc_cv_test/Measurements/Power and angle calculations/discrete low pass filter2/q rounder1 ==
  in : Inport
  Gain9 : Gain  Gain=2^-q
  Idealized ADC quantizer : simulink_extras/Additional Discrete/Idealized ADC quantizer  NumberOfConverterBits=32  Vmin=-range  Vmax=range  OutputDataType=double  OutputNegativeValues=on
  out : Outport
  wires:
  in/1 -> Idealized ADC quantizer/1
  Idealized ADC quantizer/1 -> Gain9/1
  Gain9/1 -> out/1

== system general_charger_2_cc_cv_test/Measurements/Power and angle calculations/discrete low pass filter2/q rounder10 ==
  in : Inport
  Gain9 : Gain  Gain=2^-q
  Idealized ADC quantizer : simulink_extras/Additional Discrete/Idealized ADC quantizer  NumberOfConverterBits=32  Vmin=-range  Vmax=range  OutputDataType=double  OutputNegativeValues=on
  out : Outport
  wires:
  in/1 -> Idealized ADC quantizer/1
  Idealized ADC quantizer/1 -> Gain9/1
  Gain9/1 -> out/1

== system general_charger_2_cc_cv_test/Measurements/Power and angle calculations/discrete low pass filter2/q rounder11 ==
  in : Inport
  Gain9 : Gain  Gain=2^-q
  Idealized ADC quantizer : simulink_extras/Additional Discrete/Idealized ADC quantizer  NumberOfConverterBits=32  Vmin=-range  Vmax=range  OutputDataType=double  OutputNegativeValues=on
  out : Outport
  wires:
  in/1 -> Idealized ADC quantizer/1
  Idealized ADC quantizer/1 -> Gain9/1
  Gain9/1 -> out/1

== system general_charger_2_cc_cv_test/Measurements/Power and angle calculations/discrete low pass filter2/q rounder12 ==
  in : Inport
  Gain9 : Gain  Gain=2^-q
  Idealized ADC quantizer : simulink_extras/Additional Discrete/Idealized ADC quantizer  NumberOfConverterBits=32  Vmin=-range  Vmax=range  OutputDataType=double  OutputNegativeValues=on
  out : Outport
  wires:
  in/1 -> Idealized ADC quantizer/1
  Idealized ADC quantizer/1 -> Gain9/1
  Gain9/1 -> out/1

== system general_charger_2_cc_cv_test/Measurements/Power and angle calculations/discrete low pass filter2/q rounder13 ==
  in : Inport
  Gain9 : Gain  Gain=2^-q
  Idealized ADC quantizer : simulink_extras/Additional Discrete/Idealized ADC quantizer  NumberOfConverterBits=32  Vmin=-range  Vmax=range  OutputDataType=double  OutputNegativeValues=on
  out : Outport
  wires:
  in/1 -> Idealized ADC quantizer/1
  Idealized ADC quantizer/1 -> Gain9/1
  Gain9/1 -> out/1

== system general_charger_2_cc_cv_test/Measurements/Power and angle calculations/discrete low pass filter2/q rounder14 ==
  in : Inport
  Gain9 : Gain  Gain=2^-q
  Idealized ADC quantizer : simulink_extras/Additional Discrete/Idealized ADC quantizer  NumberOfConverterBits=32  Vmin=-range  Vmax=range  OutputDataType=double  OutputNegativeValues=on
  out : Outport
  wires:
  in/1 -> Idealized ADC quantizer/1
  Idealized ADC quantizer/1 -> Gain9/1
  Gain9/1 -> out/1

== system general_charger_2_cc_cv_test/Measurements/Power and angle calculations/discrete low pass filter2/q rounder15 ==
  in : Inport
  Gain9 : Gain  Gain=2^-q
  Idealized ADC quantizer : simulink_extras/Additional Discrete/Idealized ADC quantizer  NumberOfConverterBits=32  Vmin=-range  Vmax=range  OutputDataType=double  OutputNegativeValues=on
  out : Outport
  wires:
  in/1 -> Idealized ADC quantizer/1
  Idealized ADC quantizer/1 -> Gain9/1
  Gain9/1 -> out/1

== system general_charger_2_cc_cv_test/Measurements/Power and angle calculations/discrete low pass filter2/q rounder16 ==
  in : Inport
  Gain9 : Gain  Gain=2^-q
  Idealized ADC quantizer : simulink_extras/Additional Discrete/Idealized ADC quantizer  NumberOfConverterBits=32  Vmin=-range  Vmax=range  OutputDataType=double  OutputNegativeValues=on
  out : Outport
  wires:
  in/1 -> Idealized ADC quantizer/1
  Idealized ADC quantizer/1 -> Gain9/1
  Gain9/1 -> out/1

== system general_charger_2_cc_cv_test/Measurements/Power and angle calculations/discrete low pass filter2/q rounder17 ==
  in : Inport
  Gain9 : Gain  Gain=2^-q
  Idealized ADC quantizer : simulink_extras/Additional Discrete/Idealized ADC quantizer  NumberOfConverterBits=32  Vmin=-range  Vmax=range  OutputDataType=double  OutputNegativeValues=on
  out : Outport
  wires:
  in/1 -> Idealized ADC quantizer/1
  Idealized ADC quantizer/1 -> Gain9/1
  Gain9/1 -> out/1

== system general_charger_2_cc_cv_test/Measurements/Power and angle calculations/discrete low pass filter2/q rounder2 ==
  in : Inport
  Gain9 : Gain  Gain=2^-q
  Idealized ADC quantizer : simulink_extras/Additional Discrete/Idealized ADC quantizer  NumberOfConverterBits=32  Vmin=-range  Vmax=range  OutputDataType=double  OutputNegativeValues=on
  out : Outport
  wires:
  in/1 -> Idealized ADC quantizer/1
  Idealized ADC quantizer/1 -> Gain9/1
  Gain9/1 -> out/1

== system general_charger_2_cc_cv_test/Measurements/Power and angle calculations/discrete low pass filter2/q rounder3 ==
  in : Inport
  Gain9 : Gain  Gain=2^-q
  Idealized ADC quantizer : simulink_extras/Additional Discrete/Idealized ADC quantizer  NumberOfConverterBits=32  Vmin=-range  Vmax=range  OutputDataType=double  OutputNegativeValues=on
  out : Outport
  wires:
  in/1 -> Idealized ADC quantizer/1
  Idealized ADC quantizer/1 -> Gain9/1
  Gain9/1 -> out/1

== system general_charger_2_cc_cv_test/Measurements/Power and angle calculations/discrete low pass filter2/q rounder4 ==
  in : Inport
  Gain9 : Gain  Gain=2^-q
  Idealized ADC quantizer : simulink_extras/Additional Discrete/Idealized ADC quantizer  NumberOfConverterBits=32  Vmin=-range  Vmax=range  OutputDataType=double  OutputNegativeValues=on
  out : Outport
  wires:
  in/1 -> Idealized ADC quantizer/1
  Idealized ADC quantizer/1 -> Gain9/1
  Gain9/1 -> out/1

== system general_charger_2_cc_cv_test/Measurements/Power and angle calculations/discrete low pass filter2/q rounder5 ==
  in : Inport
  Gain9 : Gain  Gain=2^-q
  Idealized ADC quantizer : simulink_extras/Additional Discrete/Idealized ADC quantizer  NumberOfConverterBits=32  Vmin=-range  Vmax=range  OutputDataType=double  OutputNegativeValues=on
  out : Outport
  wires:
  in/1 -> Idealized ADC quantizer/1
  Idealized ADC quantizer/1 -> Gain9/1
  Gain9/1 -> out/1

== system general_charger_2_cc_cv_test/Measurements/Power and angle calculations/discrete low pass filter2/q rounder6 ==
  in : Inport
  Gain9 : Gain  Gain=2^-q
  Idealized ADC quantizer : simulink_extras/Additional Discrete/Idealized ADC quantizer  NumberOfConverterBits=32  Vmin=-range  Vmax=range  OutputDataType=double  OutputNegativeValues=on
  out : Outport
  wires:
  in/1 -> Idealized ADC quantizer/1
  Idealized ADC quantizer/1 -> Gain9/1
  Gain9/1 -> out/1

== system general_charger_2_cc_cv_test/Measurements/Power and angle calculations/discrete low pass filter2/q rounder7 ==
  in : Inport
  Gain9 : Gain  Gain=2^-q
  Idealized ADC quantizer : simulink_extras/Additional Discrete/Idealized ADC quantizer  NumberOfConverterBits=32  Vmin=-range  Vmax=range  OutputDataType=double  OutputNegativeValues=on
  out : Outport
  wires:
  in/1 -> Idealized ADC quantizer/1
  Idealized ADC quantizer/1 -> Gain9/1
  Gain9/1 -> out/1

== system general_charger_2_cc_cv_test/Measurements/Power and angle calculations/discrete low pass filter2/q rounder8 ==
  in : Inport
  Gain9 : Gain  Gain=2^-q
  Idealized ADC quantizer : simulink_extras/Additional Discrete/Idealized ADC quantizer  NumberOfConverterBits=32  Vmin=-range  Vmax=range  OutputDataType=double  OutputNegativeValues=on
  out : Outport
  wires:
  in/1 -> Idealized ADC quantizer/1
  Idealized ADC quantizer/1 -> Gain9/1
  Gain9/1 -> out/1

== system general_charger_2_cc_cv_test/Measurements/Power and angle calculations/discrete low pass filter2/q rounder9 ==
  in : Inport
  Gain9 : Gain  Gain=2^-q
  Idealized ADC quantizer : simulink_extras/Additional Discrete/Idealized ADC quantizer  NumberOfConverterBits=32  Vmin=-range  Vmax=range  OutputDataType=double  OutputNegativeValues=on
  out : Outport
  wires:
  in/1 -> Idealized ADC quantizer/1
  Idealized ADC quantizer/1 -> Gain9/1
  Gain9/1 -> out/1

== system general_charger_2_cc_cv_test/Measurements/THD/RMS1/PI3 ==
  in : Inport
  Add1 : Sum
  Add2 : Sum
  Ki : Gain  Gain=ki
  Kp : Gain  Gain=kp
  Tappe : simulink/Discrete/Tapped Delay  vinit=0.0  samptime=Ts_pi  NumDelays=1  DelayOrder=Oldest  includeCurrent=off
  Ts : Gain  Gain=Ts_pi
  integral saturation : Saturate  UpperLimit=int_sat_up  LowerLimit=int_sat_low  SampleTime=Ts_pi
  pi controller saturation : Saturate  UpperLimit=pi_sat_up  LowerLimit=pi_sat_low  SampleTime=Ts_pi
  out : Outport
  wires:
  Ts/1 -> Ki/1
  in/1 -> Kp/1, Ts/1  "vdc_error"
  Add1/1 -> integral saturation/1  "vdc_int_pi"
  Kp/1 -> Add2/2  "vdc_kp_pi"
  pi controller saturation/1 -> out/1
  Tappe/1 -> Add1/1
  Add2/1 -> pi controller saturation/1  "vdc_pi"
  Ki/1 -> Add1/2
  integral saturation/1 -> Add2/1, Tappe/1

== system general_charger_2_cc_cv_test/Measurements/THD/RMS4/PI3 ==
  in : Inport
  Add1 : Sum
  Add2 : Sum
  Ki : Gain  Gain=ki
  Kp : Gain  Gain=kp
  Tappe : simulink/Discrete/Tapped Delay  vinit=0.0  samptime=Ts_pi  NumDelays=1  DelayOrder=Oldest  includeCurrent=off
  Ts : Gain  Gain=Ts_pi
  integral saturation : Saturate  UpperLimit=int_sat_up  LowerLimit=int_sat_low  SampleTime=Ts_pi
  pi controller saturation : Saturate  UpperLimit=pi_sat_up  LowerLimit=pi_sat_low  SampleTime=Ts_pi
  out : Outport
  wires:
  Ts/1 -> Ki/1
  in/1 -> Kp/1, Ts/1  "vdc_error"
  Add1/1 -> integral saturation/1  "vdc_int_pi"
  Kp/1 -> Add2/2  "vdc_kp_pi"
  pi controller saturation/1 -> out/1
  Tappe/1 -> Add1/1
  Add2/1 -> pi controller saturation/1  "vdc_pi"
  Ki/1 -> Add1/2
  integral saturation/1 -> Add2/1, Tappe/1

== system general_charger_2_cc_cv_test/Measurements/THD/discrete low pass filter1/Ad(1,1) ==
  in : Inport
  Constant1 : Constant  Value=variable
  Product1 : Product
  q rounder16 : Subsystem  mask{q=nQ, range=maxRange}
      mask prompts: q "q value"; range "q range"
  out : Outport
  wires:
  q rounder16/1(out) -> Product1/1
  Constant1/1 -> q rounder16/1(in)
  Product1/1 -> out/1
  in/1 -> Product1/2

== system general_charger_2_cc_cv_test/Measurements/THD/discrete low pass filter1/Ad(1,2) ==
  in : Inport
  Constant1 : Constant  Value=variable
  Product1 : Product
  q rounder16 : Subsystem  mask{q=nQ, range=maxRange}
      mask prompts: q "q value"; range "q range"
  out : Outport
  wires:
  q rounder16/1(out) -> Product1/1
  Constant1/1 -> q rounder16/1(in)
  Product1/1 -> out/1
  in/1 -> Product1/2

== system general_charger_2_cc_cv_test/Measurements/THD/discrete low pass filter1/Ad(1,3) ==
  in : Inport
  Constant1 : Constant  Value=variable
  Product1 : Product
  Scope1 : Scope  NumInputPorts=2
      settings: YMin=-5~-5  YMax=5~5
  q rounder16 : Subsystem  mask{q=nQ, range=maxRange}
      mask prompts: q "q value"; range "q range"
  out : Outport
  wires:
  q rounder16/1(out) -> Product1/1, Scope1/2
  Constant1/1 -> Scope1/1, q rounder16/1(in)
  Product1/1 -> out/1
  in/1 -> Product1/2
